simulink model "plant_Model"  (R2020a)
settings: Solver=VariableStepAuto  StartTime=0.0  StopTime=10.0  RelTol=1e-3
undefined symbols (not defined in the file or in its folder): b, m
settings Model: DataDictionary=cruise_ControlParameter.sldd  Creator=INDRAJIT MARATHE  LastModifiedBy=INDRAJIT MARATHE

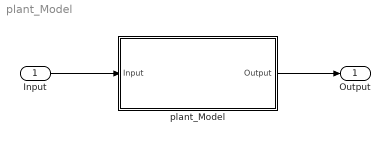
== system plant_Model ==
  " Input" : Inport
  plant_Model : Subsystem  TreatAsAtomicUnit=on
  " Output" : Outport
  wires:
  " Input"/1 -> plant_Model/1(" Input")
  plant_Model/1(" Output") -> " Output"/1

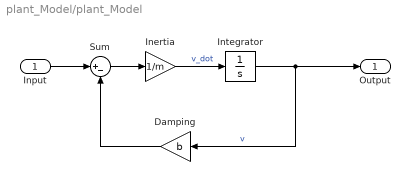
== system plant_Model/plant_Model ==
  " Input" : Inport
  " Integrator" : Integrator
  " Sum" : Sum  Inputs=|+-
  Damping : Gain  Gain=b
  Inertia : Gain  Gain=1/m
  " Output" : Outport
  wires:
  Inertia/1 -> " Integrator"/1  "v_dot"
  " Input"/1 -> " Sum"/1
  " Sum"/1 -> Inertia/1
  " Integrator"/1 -> " Output"/1, Damping/1  "v"
  Damping/1 -> " Sum"/2
